simulink model "SendRandomStimXpcTarget"  (R2016b)
settings: Solver=FixedStepDiscrete  StartTime=0.0  StopTime=inf  FixedStep=sCoreParams.core.stepPeriod  RelTol=1e-3  EnableMultiTasking=on
values from neighbouring files (symbols this model uses):
  sCoreParams = InitCoreParams_Dependent(sCoreParams)    [initializationScript.m]
libraries: slrtlib x6
settings Model: Creator=rzelmann  LastModifiedBy=rzelmann
settings SolverCC: EnableConcurrentExecution=on  ConcurrentTasks=on
settings DataIOCC: SaveFormat=StructureWithTime
settings OptimizationCC: DefaultParameterBehavior=Inlined  EfficientFloat2IntCast=on  LifeSpan=inf
settings DebuggingCC: UniqueDataStoreMsg=error  StrictBusMsg=ErrorOnBusTreatedAsVector  SFUnexpectedBacktrackingDiag=warning  SFNoUnconditionalDefaultTransitionDiag=warning  SFExecutionAtInitializationDiag=none
settings HardwareCC: ProdBitPerPointer=32  ProdBitPerSizeT=32  ProdBitPerPtrDiffT=32  ProdLargestAtomicFloat=None  ProdWordSize=32  ProdLongLongMode=on  ProdHWDeviceType=Generic->32-bit x86 compatible
settings ModelReferenceCC: ModelReferenceNumInstancesAllowed=Single
settings RTWCC: SystemTargetFile=slrt.tlc  TLCOptions="-axPCMaxOverloads=30            -axPCOverLoadLen=2 -axPCStartupFlag=5"  TemplateMakefile=slrt_default_tmf  Description=Simulink Real-Time  RTWCompilerOptimization=on
settings CodeAppCC: MaxIdLength=63
settings ConfigComp: CovMetricSettings=dw  CovHtmlReporting=on  CovSaveCumulativeToWorkspaceVar=on  CovSaveSingleToWorkspaceVar=on  CovExternalEMLEnable=off

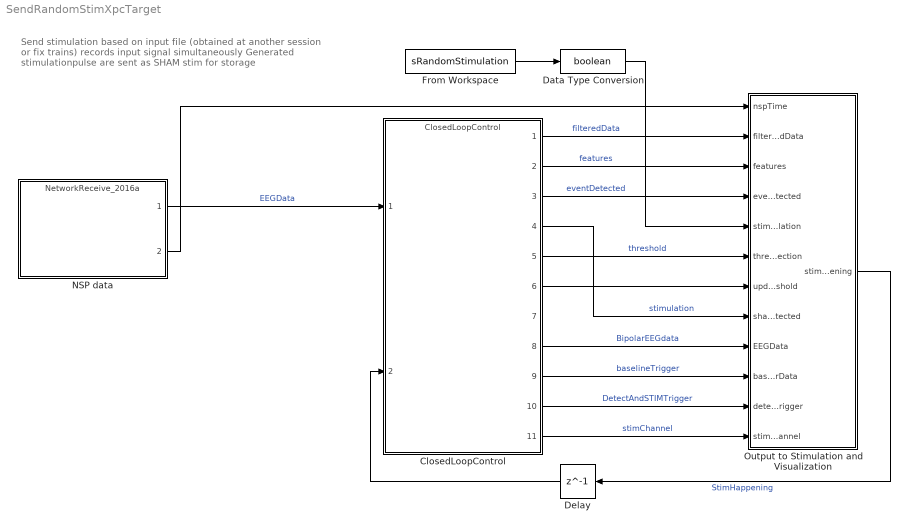
== system SendRandomStimXpcTarget ==
  note: Send stimulation based on input file
      | (obtained at another session or fix trains)
      | records input signal simultaneously
      |
      | Generated stimulationpulse are sent as SHAM stim for storage
  ClosedLoopControl : ModelReference  ModelNameDialog=ClosedLoopControl  SimulationMode=Normal  ModelReferenceVersion=1.610
  Data Type Conversion : DataTypeConversion  OutDataTypeStr=boolean
  Delay : Delay  DelayLength=1  InitialCondition=0  InputProcessing=Columns as channels (frame based)  SampleTime=sCoreParams.core.stepPeriod
  From Workspace : FromWorkspace  VariableName=sRandomStimulation  SampleTime=sCoreParams.core.stepPeriod  Interpolate=off  OutputAfterFinalValue=Cyclic repetition
  NSP data : ModelReference  ModelNameDialog=NetworkReceive_2016a.slx  SimulationMode=Normal  ModelReferenceVersion=1.183
  Output to Stimulation and Visualization : Subsystem
  wires:
  Output to Stimulation and Visualization/1(stimHappening) -> Delay/1  "StimHappening"
  NSP data/1 -> ClosedLoopControl/1  "EEGData"
  ClosedLoopControl/1 -> Output to Stimulation and Visualization/2(filteredData)  "filteredData"
  NSP data/2 -> Output to Stimulation and Visualization/1(nspTime)
  ClosedLoopControl/2 -> Output to Stimulation and Visualization/3(features)  "features"
  ClosedLoopControl/3 -> Output to Stimulation and Visualization/4(eventDetected)  "eventDetected"
  ClosedLoopControl/5 -> Output to Stimulation and Visualization/6(thresholdUsedInDetection)  "threshold"
  ClosedLoopControl/6 -> Output to Stimulation and Visualization/7(updatingThreshold)
  ClosedLoopControl/8 -> Output to Stimulation and Visualization/9(EEGData)  "BipolarEEGdata"
  ClosedLoopControl/9 -> Output to Stimulation and Visualization/10(baselineTriggerData)  "baselineTrigger"
  ClosedLoopControl/10 -> Output to Stimulation and Visualization/11(detectionStimTrigger)  "DetectAndSTIMTrigger"
  Delay/1 -> ClosedLoopControl/2
  ClosedLoopControl/11 -> Output to Stimulation and Visualization/12(stimChannel)  "stimChannel"
  From Workspace/1 -> Data Type Conversion/1
  ClosedLoopControl/4 -> Output to Stimulation and Visualization/8(shamDetected)  "stimulation"
  Data Type Conversion/1 -> Output to Stimulation and Visualization/5(stimulation)

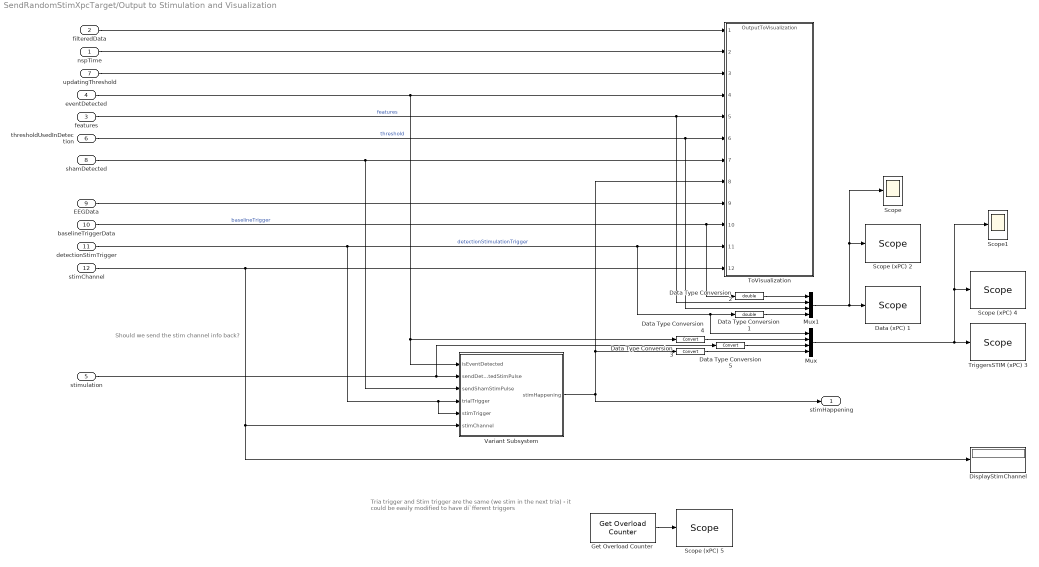
== system SendRandomStimXpcTarget/Output to Stimulation and Visualization ==
  note: Should we send the stim channel info back?
  note: Tria trigger and Stim trigger are the same (we stim in the next tria)
      | - it could be easily modified to have di`fferent triggers
  nspTime : Inport
  filteredData : Inport  Port=2
  features : Inport  Port=3
  eventDetected : Inport  Port=4
  stimulation : Inport  Port=5
  thresholdUsedInDetection : Inport  Port=6
  updatingThreshold : Inport  Port=7
  shamDetected : Inport  Port=8
  EEGData : Inport  Port=9
  baselineTriggerData : Inport  Port=10  OutDataTypeStr=int32
  detectionStimTrigger : Inport  Port=11  OutDataTypeStr=int32
  stimChannel : Inport  Port=12
  Data (xPC) 1 : slrtlib/Displays and Logging/Scope   scopeno=1  scopetype=Target  autostart=on  viewmode=Graphical redraw  formatstr='%15.6f'  grid=on  ylimits=[0,0]  nosamples=1000  noprepostsamples=0  interleave=1  triggermode=FreeRun  triggersignal=1  trigsignalfromport=on  triggerlevel=0.0  triggerslope=Rising  triggerscope=1  triggersample=0  filename=data.dat  mode=Lazy  writesize=512  autorestart=off  dynamicfilemode=off  maxwritefilesize=512*1024^2
  Data Type Conversion1 : DataTypeConversion  OutDataTypeStr=double
  Data Type Conversion2 : DataTypeConversion  OutDataTypeStr=double
  Data Type Conversion3 : DataTypeConversion
  Data Type Conversion4 : DataTypeConversion
  Data Type Conversion5 : DataTypeConversion
  DisplayStimChannel : Display
  "Get Overload Counter " : slrtlib/Target Management/Execution Parameters/Get Overload Counter   ts=sCoreParams.core.stepPeriod
  Mux : Mux
  Mux1 : Mux
  Scope : Scope
  Scope (xPC) 2 : slrtlib/Displays and Logging/Scope   scopeno=2  scopetype=File  autostart=on  viewmode=Graphical redraw  formatstr='%15.6f'  grid=on  ylimits=[0,0]  nosamples=1000  noprepostsamples=-10  interleave=1  triggermode=FreeRun  triggersignal=1  trigsignalfromport=on  triggerlevel=0.0  triggerslope=Rising  triggerscope=1  triggersample=0  filename=featTh.dat  mode=Lazy  writesize=512  autorestart=off  dynamicfilemode=off  maxwritefilesize=512*1024^2
  Scope (xPC) 4 : slrtlib/Displays and Logging/Scope   scopeno=4  scopetype=File  autostart=on  viewmode=Graphical redraw  formatstr='%15.6f'  grid=on  ylimits=[0,0]  nosamples=1000  noprepostsamples=-10  interleave=1  triggermode=FreeRun  triggersignal=1  trigsignalfromport=on  triggerlevel=0.0  triggerslope=Rising  triggerscope=1  triggersample=0  filename=detStim.dat  mode=Lazy  writesize=512  autorestart=off  dynamicfilemode=off  maxwritefilesize=512*1024^2
  Scope (xPC) 5 : slrtlib/Displays and Logging/Scope   scopeno=5  scopetype=Target  autostart=on  viewmode=Graphical redraw  formatstr='%15.6f'  grid=on  ylimits=[0,0]  nosamples=1000  noprepostsamples=0  interleave=1  triggermode=FreeRun  triggersignal=1  trigsignalfromport=on  triggerlevel=0.0  triggerslope=Rising  triggerscope=1  triggersample=0  filename=data.dat  mode=Lazy  writesize=512  autorestart=off  dynamicfilemode=off  maxwritefilesize=512*1024^2
  Scope1 : Scope
  ToVisualization : ModelReference  ModelNameDialog=OutputToVisualization  SimulationMode=Normal  ModelReferenceVersion=1.227
  TriggersSTIM (xPC) 3 : slrtlib/Displays and Logging/Scope   scopeno=3  scopetype=Target  autostart=on  viewmode=Graphical redraw  formatstr='%15.6f'  grid=on  ylimits=[0,0]  nosamples=1000  noprepostsamples=0  interleave=1  triggermode=FreeRun  triggersignal=1  trigsignalfromport=on  triggerlevel=0.0  triggerslope=Rising  triggerscope=1  triggersample=0  filename=data.dat  mode=Lazy  writesize=512  autorestart=off  dynamicfilemode=off  maxwritefilesize=512*1024^2
  Variant Subsystem : Subsystem  Variant=on
  stimHappening : Outport
  wires:
  updatingThreshold/1 -> ToVisualization/3
  shamDetected/1 -> Variant Subsystem/3(sendShamStimPulse), ToVisualization/7
  filteredData/1 -> ToVisualization/1
  EEGData/1 -> ToVisualization/9
  eventDetected/1 -> ToVisualization/4, Data Type Conversion4/1, Variant Subsystem/1(isEventDetected)
  Variant Subsystem/1(stimHappening) -> ToVisualization/8, Data Type Conversion3/1, stimHappening/1
  stimulation/1 -> Data Type Conversion5/1, Variant Subsystem/2(sendDetectedStimPulse)
  features/1 -> Mux1/2, ToVisualization/5  "features"
  thresholdUsedInDetection/1 -> Mux1/3, ToVisualization/6  "threshold"
  nspTime/1 -> ToVisualization/2
  Data Type Conversion3/1 -> Mux/4
  Data Type Conversion4/1 -> Mux/2
  Mux1/1 -> Scope/1, Scope (xPC) 2/1, Data (xPC) 1/1
  Mux/1 -> Scope1/1, Scope (xPC) 4/1, TriggersSTIM (xPC) 3/1
  Data Type Conversion5/1 -> Mux/3
  baselineTriggerData/1 -> Data Type Conversion2/1, ToVisualization/10  "baselineTrigger"
  Data Type Conversion2/1 -> Mux1/1
  "Get Overload Counter "/1 -> Scope (xPC) 5/1
  detectionStimTrigger/1 -> Mux/1, Data Type Conversion1/1, ToVisualization/11, Variant Subsystem/5(stimTrigger), Variant Subsystem/4(trialTrigger)  "detectionStimulationTrigger"
  Data Type Conversion1/1 -> Mux1/4
  stimChannel/1 -> Variant Subsystem/6(stimChannel), DisplayStimChannel/1, ToVisualization/12

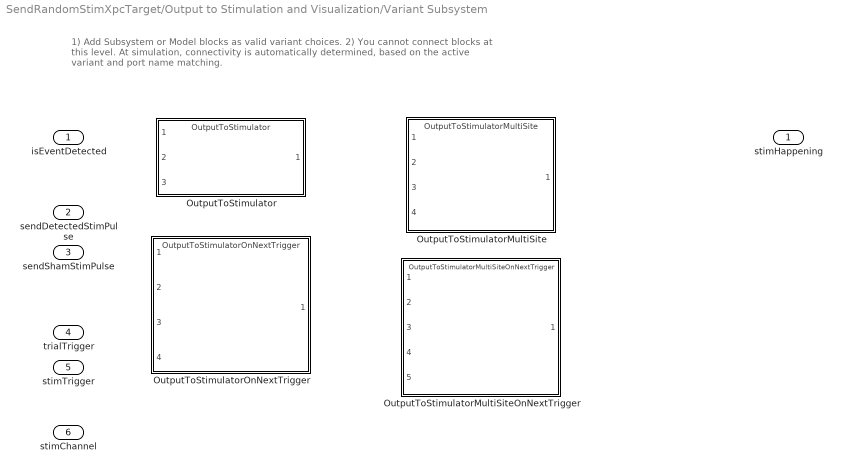
== system SendRandomStimXpcTarget/Output to Stimulation and Visualization/Variant Subsystem ==
  note: 1) Add Subsystem or Model blocks as valid variant choices.
      | 2) You cannot connect blocks at this level. At simulation, connectivity is automatically
      | determined, based on the active variant and port name matching.
  isEventDetected : Inport
  sendDetectedStimPulse : Inport  Port=2
  sendShamStimPulse : Inport  Port=3
  trialTrigger : Inport  Port=4
  stimTrigger : Inport  Port=5  OutDataTypeStr=int32
  stimChannel : Inport  Port=6  OutDataTypeStr=int32
  OutputToStimulator : ModelReference  ModelNameDialog=OutputToStimulator  SimulationMode=Normal  VariantControl=variantParams_STIMULATION_REALTIME  ModelReferenceVersion=1.29
  OutputToStimulatorMultiSite : ModelReference  ModelNameDialog=OutputToStimulatorMultiSite.slx  SimulationMode=Normal  VariantControl=variantParams_STIMULATION_MULTISITE_REALTIME  ModelReferenceVersion=1.44
  OutputToStimulatorMultiSiteOnNextTrigger : ModelReference  ModelNameDialog=OutputToStimulatorMultiSiteOnNextTrigger.slx  SimulationMode=Normal  VariantControl=variantParams_STIMULATION_MULTISITE_NEXTTRIGGER  ModelReferenceVersion=1.60
  OutputToStimulatorOnNextTrigger : ModelReference  ModelNameDialog=OutputToStimulatorOnNextTrigger  SimulationMode=Normal  VariantControl=variantParams_STIMULATION_ONNEXTTRIGGER  ModelReferenceVersion=1.42
  stimHappening : Outport
